simulink model "kp_ki_kd"  (R2023a)
settings: Solver=VariableStepAuto  StartTime=0.0  StopTime=10.0  RelTol=1e-3
settings Model: Creator=TUBA  LastModifiedBy=TUBA

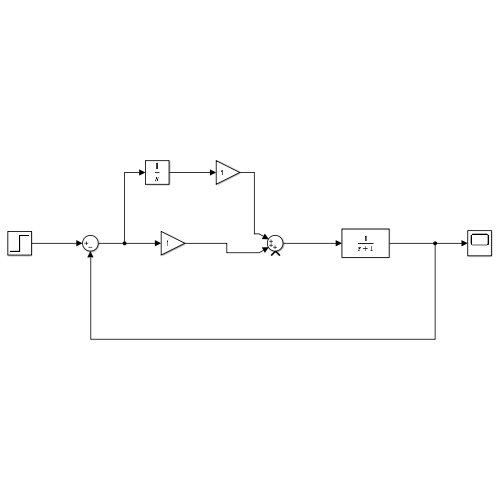
[thumbnail: Simulink's stored preview of the top-level diagram]
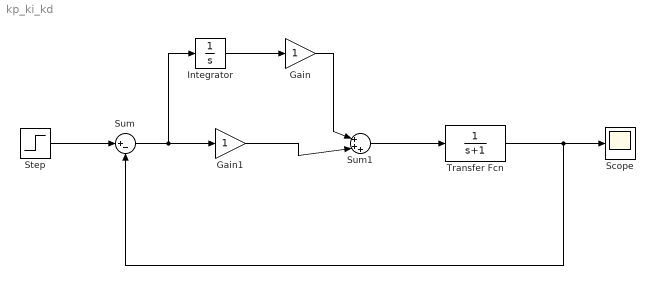
== system kp_ki_kd ==
  Gain : Gain
  Gain1 : Gain
  Integrator : Integrator
  Scope : Scope
  Step : Step  SampleTime=0
  Sum : Sum  Inputs=|+-
  Sum1 : Sum  Inputs=|+++
  Transfer Fcn : TransferFcn  Denominator=[1 1]
  wires:
  Transfer Fcn/1 -> Sum/2, Scope/1
  Integrator/1 -> Gain/1
  Step/1 -> Sum/1
  Sum/1 -> Integrator/1, Gain1/1
  Sum1/1 -> Transfer Fcn/1
  Gain/1 -> Sum1/1
  Gain1/1 -> Sum1/2
